simulink model "HEasy_export"  (Simulink 7.9)
settings: Solver=ode45  StartTime=0.0  StopTime=10.0  RelTol=1e-3
settings Model: Creator=boakes  LastModifiedBy=boakes

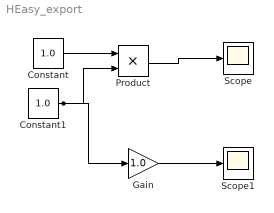
== system HEasy_export ==
  Constant : Constant  Value=1.0
  Constant1 : Constant  Value=1.0
  Gain : Gain  Gain=1.0
  Product : Product  RndMeth=Zero
  Scope : Scope
      settings: SaveName=ScopeData2
  Scope1 : Scope
      settings: SaveName=ScopeData2
  wires:
  Product/1 -> Scope/1
  Constant/1 -> Product/1
  Gain/1 -> Scope1/1
  Constant1/1 -> Gain/1, Product/2
